simulink model "kapitsa_pendulum"  (R2023b)
settings: Solver=VariableStepAuto  StartTime=0.0  StopTime=10.0  MaxStep=1e-2  RelTol=1e-3
libraries: simulink_extras x3
settings Model: Creator=B03-401  LastModifiedBy=B03-401

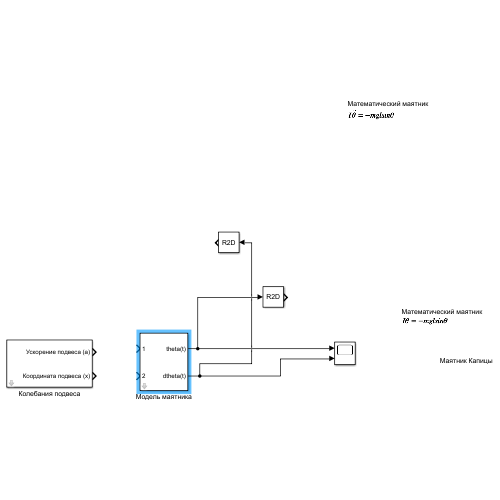
[thumbnail: Simulink's stored preview of the top-level diagram]
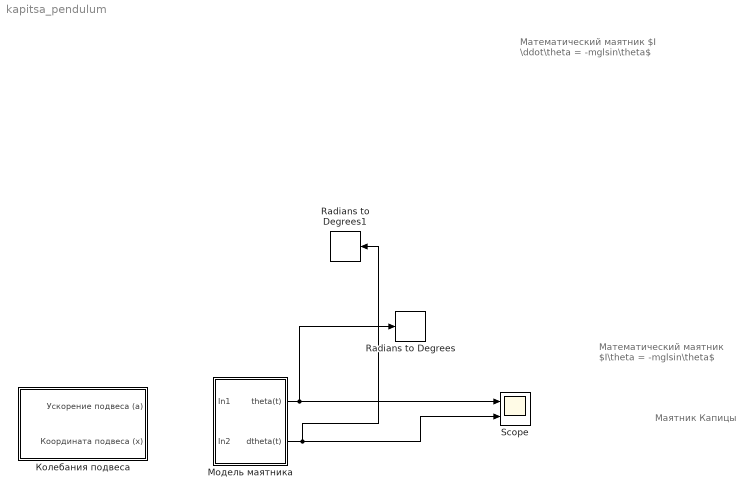
== system kapitsa_pendulum ==
  note: Маятник Капицы
  note: Математический маятник
      | $I\theta = -mglsin\theta$
  note: Математический маятник
      | $I \ddot\theta = -mglsin\theta$
  Radians to Degrees : simulink_extras/Transformations/Radians to Degrees
  Radians to Degrees1 : simulink_extras/Transformations/Radians to Degrees
  Scope : Scope  NumInputPorts=2
  Колебания подвеса : Subsystem  mask{A=1, v=1}
      mask prompts: A "Амплитуда (м)"; v "Частота (Гц)"
  Модель маятника : Subsystem  mask{m=0, L=0, g=0, startDegree=0, b=10}
      mask prompts: m "Масса, кг"; L "Длина, м"; g "Уск. своб. пад., м/с^2"; startDegree "Градусы"; b "Диссипативный член"
  wires:
  Модель маятника/1(theta(t)) -> Radians to Degrees/1, Scope/1
  Модель маятника/2(dtheta(t)) -> Radians to Degrees1/1, Scope/2

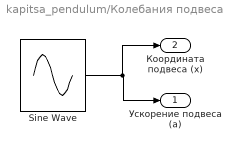
== system kapitsa_pendulum/Колебания подвеса ==
  Sine Wave : Sin  Frequency=1*2*pi  SampleTime=0
  Ускорение подвеса (a) : Outport
  Координата подвеса (x) : Outport  Port=2
  wires:
  Sine Wave/1 -> Координата подвеса (x)/1, Ускорение подвеса (a)/1

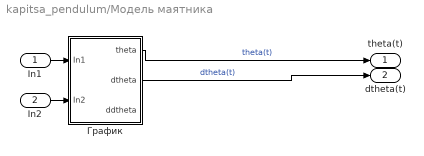
== system kapitsa_pendulum/Модель маятника ==
  In1 : Inport
  In2 : Inport  Port=2
  График : Subsystem  mask{m=1, L=1, g=9.8, startDegree=30}
      mask prompts: m "mass"; L "length"
  theta(t) : Outport
  dtheta(t) : Outport  Port=2
  wires:
  График/1(theta) -> theta(t)/1  "theta(t)"
  График/2(dtheta) -> dtheta(t)/1  "dtheta(t)"
  In1/1 -> График/1(In1)
  In2/1 -> График/2(In2)

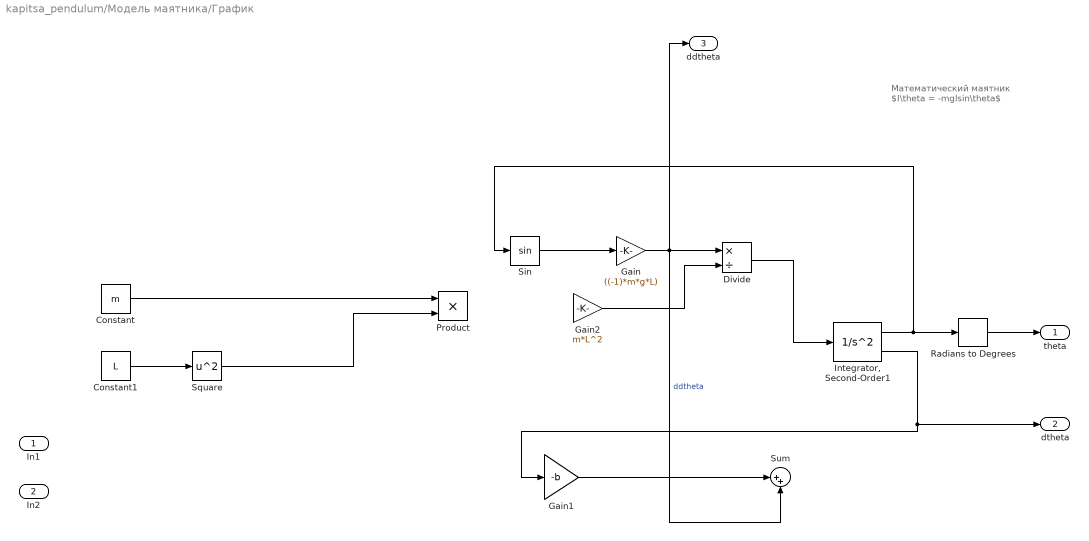
== system kapitsa_pendulum/Модель маятника/График ==
  note: Математический маятник
      | $I\theta = -mglsin\theta$
  In1 : Inport
  In2 : Inport  Port=2
  Constant : Constant  Value=m
  Constant1 : Constant  Value=L
  Divide : Product  Inputs=*/
  Gain : Gain  Gain=((-1)*m*g*L)
  Gain1 : Gain  Gain=-b
  Gain2 : Gain  Gain=m*L^2
  "Integrator, Second-Order1" : SecondOrderIntegrator  ICX=deg2rad(startDegree)
  Product : Product
  Radians to Degrees : simulink_extras/Transformations/Radians to Degrees
  Sin : Trigonometry
  Square : Math  Operator=square
  Sum : Sum  Inputs=|++
  theta : Outport
  dtheta : Outport  Port=2
  ddtheta : Outport  Port=3
  wires:
  "Integrator, Second-Order1"/2 -> Gain1/1, dtheta/1
  "Integrator, Second-Order1"/1 -> Sin/1, Radians to Degrees/1
  Constant/1 -> Product/1
  Constant1/1 -> Square/1
  Square/1 -> Product/2
  Sin/1 -> Gain/1
  Gain/1 -> Sum/2, ddtheta/1, Divide/1  "ddtheta"
  Divide/1 -> "Integrator, Second-Order1"/1
  Radians to Degrees/1 -> theta/1
  Gain1/1 -> Sum/1
  Gain2/1 -> Divide/2
